simulink model "mbdo_full"  (Simulink 9.0)
settings: Solver=FixedStepDiscrete  StartTime=0  StopTime=simulationDuration  FixedStep=dt  MaxStep=0.001  RelTol=1e-3  EnableMultiTasking=on
InitFcn:
  | mbdoParams
StartFcn:
  | mbdoParams
values from neighbouring files (symbols this model uses):
  desBasePos = basePoseW    [mbdoParams.m]
undefined symbols (not defined in the file or in its folder): adjustEulerRates, computeFullDynamics, computeGrfs, computeVcross, DiscIntNeverNeededParam, Dj, dt, Gain, Ic, Kj, mapWrenchToTorques, q_des, simulinkAnim, updateStates
undefined symbols (not defined in the file): inputForce, Kdang, Kdlin, Kpang, Kplin
libraries: simulink x2
settings Model: SuppressorTable=22 serialization::archive 11 0 6 0 0 0 11 0  Creator=mfocchi  LastModifiedBy=nikhil
settings DataIOCC: LimitDataPoints=on
settings OptimizationCC: ExpressionDepthLimit=2147483647  InitFltsAndDblsToZero=on
settings DebuggingCC: SolverPrmCheckMsg=warning  FcnCallInpInsideContextMsg=warning  StateNameClashWarn=warning
settings GRTTargetCC: CombineOutputUpdateFcns=off  GRTInterface=on

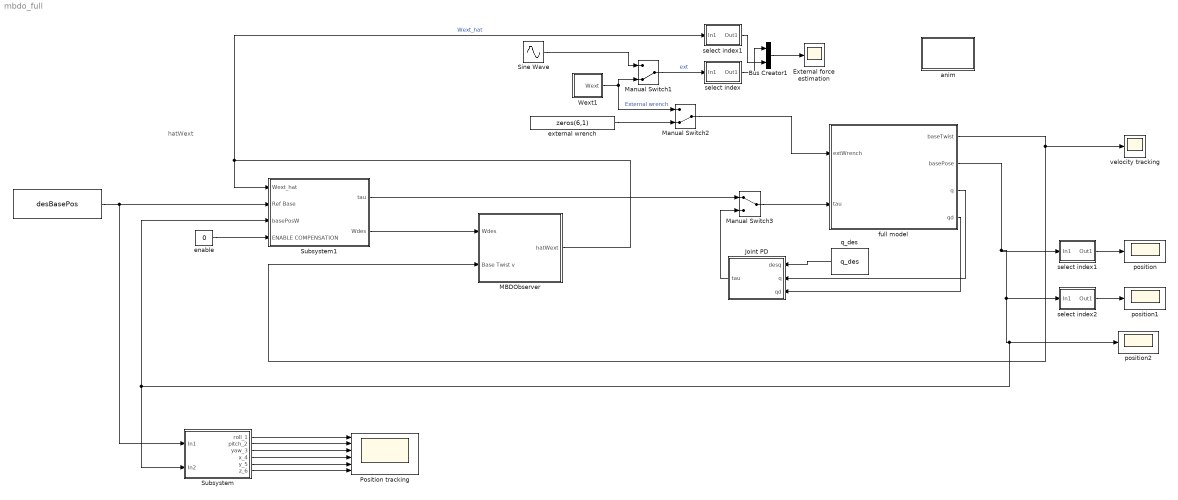
== system mbdo_full ==
  note: hatWext
  " " : Constant  Value=desBasePos
  Bus Creator1 : BusCreator  Inputs=2
  External force estimation : Scope
  Joint PD : Subsystem
  MBDObserver : Subsystem
  Manual Switch1 : ManualSwitch  CurrentSetting=0
  Manual Switch2 : ManualSwitch  CurrentSetting=0
  Manual Switch3 : ManualSwitch
  Position tracking : Scope  NumInputPorts=6
  Sine Wave : Sin  Amplitude=100  Frequency=2*pi*5  SampleTime=0
  Subsystem : Subsystem
  Subsystem1 : Subsystem
  Wext1 : Subsystem  mask{input=inputForce, fext=200, step_time=3}
  anim : Subsystem
  enable : Constant  Value=0
  external wrench : Constant  Value=zeros(6,1)
  full model : Subsystem
  position : Scope
  position1 : Scope
  position2 : Scope
  q_des : Constant  Value=q_des
  select index : Subsystem  mask{input=inputForce}
  select index1 : Subsystem  mask{input=6}
  "select index1 " : Subsystem  mask{input=inputForce}
  select index2 : Subsystem  mask{input=2}
  velocity tracking : Scope
  wires:
  " "/1 -> Subsystem/1(In1), Subsystem1/2(Ref Base)
  Bus Creator1/1 -> External force estimation/1
  select index/1(Out1) -> Bus Creator1/1
  "select index1 "/1(Out1) -> Bus Creator1/2
  Manual Switch1/1 -> select index/1(In1)  "ext"
  Wext1/1(Wext) -> Manual Switch1/2, Manual Switch2/1  "External wrench"
  Sine Wave/1 -> Manual Switch1/1
  full model/2(basePose) -> Subsystem1/3(basePosW), Subsystem/2(In2), position2/1, select index2/1(In1), select index1/1(In1)
  Subsystem/1(roll_1) -> Position tracking/1
  Subsystem/2(pitch_2) -> Position tracking/2
  Subsystem/3(yaw_3) -> Position tracking/3
  Subsystem/4(x_4) -> Position tracking/4
  Subsystem/5(y_5) -> Position tracking/5
  Subsystem/6(z_6) -> Position tracking/6
  MBDObserver/1("hatWext ") -> "select index1 "/1(In1), Subsystem1/1(Wext_hat)  "Wext_hat"
  full model/1(baseTwist) -> MBDObserver/2(Base Twist v), velocity tracking/1
  select index1/1(Out1) -> position/1
  external wrench/1 -> Manual Switch2/2
  Manual Switch2/1 -> full model/1(extWrench)
  Manual Switch3/1 -> full model/2(tau)
  q_des/1 -> Joint PD/1(desq)
  full model/3(q) -> Joint PD/2(q)
  Joint PD/1(tau) -> Manual Switch3/2
  select index2/1(Out1) -> position1/1
  full model/4(qd) -> Joint PD/3(qd)
  Subsystem1/2(Wdes) -> MBDObserver/1(Wdes)
  Subsystem1/1(tau) -> Manual Switch3/1
  enable/1 -> Subsystem1/4(ENABLE COMPENSATION)

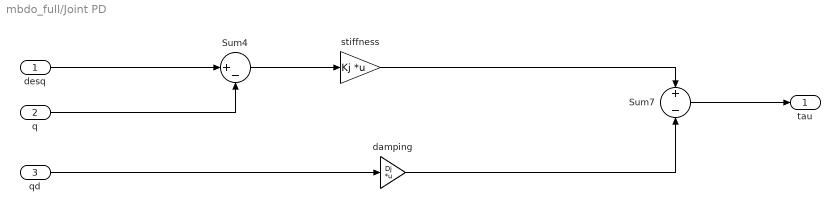
== system mbdo_full/Joint PD ==
  desq : Inport
  q : Inport  Port=2
  qd : Inport  Port=3
  Sum4 : Sum  Inputs=|+-
  Sum7 : Sum  Inputs=+|-
  damping : Gain  Gain=Dj  Multiplication=Matrix(K*u)
  stiffness : Gain  Gain=Kj  Multiplication=Matrix(K*u)
  tau : Outport
  wires:
  q/1 -> Sum4/2
  desq/1 -> Sum4/1
  Sum7/1 -> tau/1
  damping/1 -> Sum7/2
  stiffness/1 -> Sum7/1
  Sum4/1 -> stiffness/1
  qd/1 -> damping/1

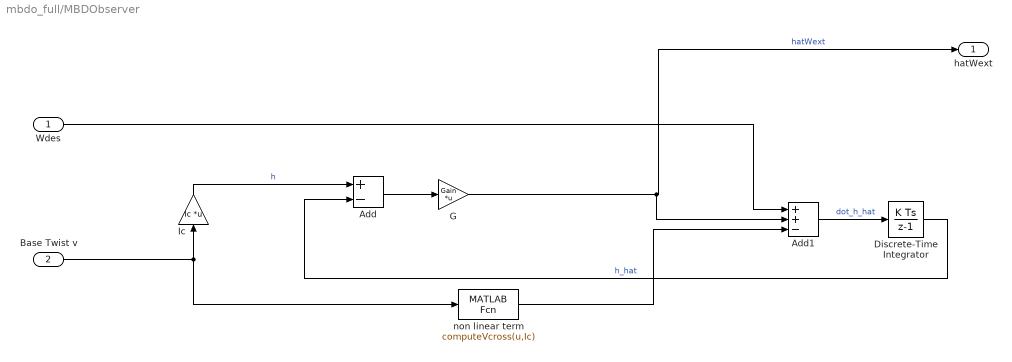
== system mbdo_full/MBDObserver ==
  Wdes : Inport
  Base Twist v : Inport  Port=2
  Add : Sum  Inputs=+-
  Add1 : Sum  Inputs=++-
  Discrete-Time Integrator : DiscreteIntegrator  InitialCondition=zeros(6,1)  InitialConditionSetting=State (most efficient)  SampleTime=dt  ICPrevOutput=DiscIntNeverNeededParam  ICPrevScaledInput=DiscIntNeverNeededParam
  G : Gain  Gain=Gain  Multiplication=Matrix(K*u)
  Ic : Gain  Gain=Ic  Multiplication=Matrix(K*u)
  non linear term : MATLABFcn  MATLABFcn=computeVcross(u,Ic)
  "hatWext " : Outport
  wires:
  G/1 -> Add1/2, "hatWext "/1  "hatWext"
  Wdes/1 -> Add1/1
  Base Twist v/1 -> non linear term/1, Ic/1
  Add/1 -> G/1
  Add1/1 -> Discrete-Time Integrator/1  "dot_h_hat"
  Ic/1 -> Add/1  "h"
  Discrete-Time Integrator/1 -> Add/2  "h_hat"
  non linear term/1 -> Add1/3

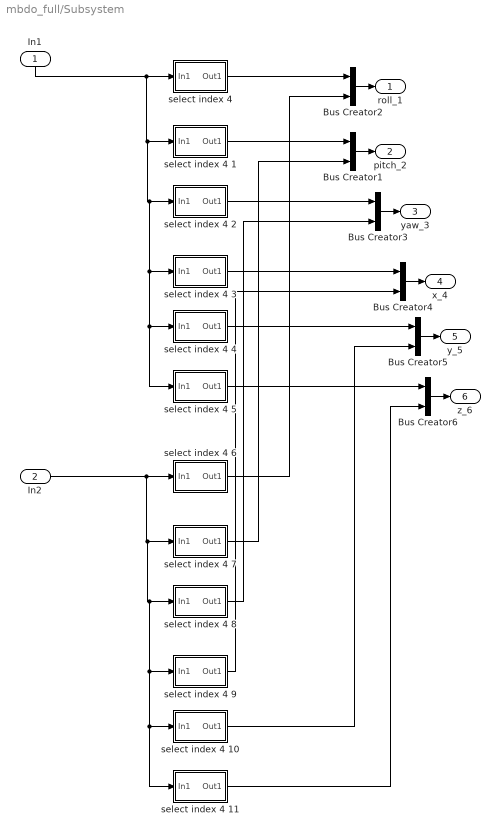
== system mbdo_full/Subsystem ==
  In1 : Inport
  In2 : Inport  Port=2
  Bus Creator{1..6} (6 alike) : BusCreator  Inputs=2
  "select index 4 " : Subsystem  mask{input=1}
  select index 4 1 : Subsystem  mask{input=2}
  select index 4 10 : Subsystem  mask{input=5}
  select index 4 11 : Subsystem  mask{input=6}
  select index 4 2 : Subsystem  mask{input=3}
  select index 4 3 : Subsystem  mask{input=4}
  select index 4 4 : Subsystem  mask{input=5}
  select index 4 5 : Subsystem  mask{input=6}
  select index 4 6 : Subsystem  mask{input=1}
  select index 4 7 : Subsystem  mask{input=2}
  select index 4 8 : Subsystem  mask{input=3}
  select index 4 9 : Subsystem  mask{input=4}
  roll_1 : Outport
  pitch_2 : Outport  Port=2
  yaw_3 : Outport  Port=3
  x_4 : Outport  Port=4
  y_5 : Outport  Port=5
  z_6 : Outport  Port=6
  wires:
  Bus Creator2/1 -> roll_1/1
  "select index 4 "/1(Out1) -> Bus Creator2/1
  In1/1 -> select index 4 5/1(In1), select index 4 4/1(In1), select index 4 3/1(In1), select index 4 2/1(In1), select index 4 1/1(In1), "select index 4 "/1(In1)
  In2/1 -> select index 4 11/1(In1), select index 4 10/1(In1), select index 4 9/1(In1), select index 4 8/1(In1), select index 4 7/1(In1), select index 4 6/1(In1)
  select index 4 6/1(Out1) -> Bus Creator2/2
  select index 4 7/1(Out1) -> Bus Creator1/2
  select index 4 1/1(Out1) -> Bus Creator1/1
  Bus Creator1/1 -> pitch_2/1
  Bus Creator3/1 -> yaw_3/1
  select index 4 8/1(Out1) -> Bus Creator3/2
  select index 4 9/1(Out1) -> Bus Creator4/2
  Bus Creator4/1 -> x_4/1
  Bus Creator5/1 -> y_5/1
  select index 4 10/1(Out1) -> Bus Creator5/2
  select index 4 11/1(Out1) -> Bus Creator6/2
  Bus Creator6/1 -> z_6/1
  select index 4 2/1(Out1) -> Bus Creator3/1
  select index 4 3/1(Out1) -> Bus Creator4/1
  select index 4 4/1(Out1) -> Bus Creator5/1
  select index 4 5/1(Out1) -> Bus Creator6/1

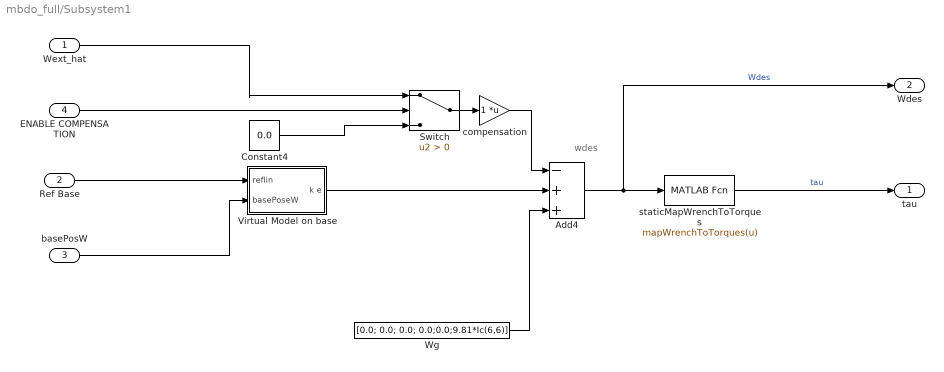
== system mbdo_full/Subsystem1 ==
  note: wdes
  Wext_hat : Inport
  Ref Base : Inport  Port=2
  basePosW : Inport  Port=3
  ENABLE COMPENSATION : Inport  Port=4
  Add4 : Sum  Inputs=-++
  Constant4 : Constant  Value=0.0
  Switch : Switch  Criteria=u2 > Threshold
  Virtual Model on base : Subsystem
  Wg : Constant  Value=[0.0; 0.0; 0.0; 0.0;0.0;9.81*Ic(6,6)]
  compensation : Gain  Multiplication=Matrix(K*u)
  staticMapWrenchToTorques : MATLABFcn  MATLABFcn=mapWrenchToTorques(u)
  tau : Outport
  Wdes : Outport  Port=2
  wires:
  basePosW/1 -> Virtual Model on base/2(basePoseW)
  Add4/1 -> Wdes/1, staticMapWrenchToTorques/1  "Wdes"
  Ref Base/1 -> Virtual Model on base/1(reflin)
  Constant4/1 -> Switch/3
  Switch/1 -> compensation/1
  Virtual Model on base/1(k e) -> Add4/2
  compensation/1 -> Add4/1
  Wg/1 -> Add4/3
  staticMapWrenchToTorques/1 -> tau/1  "tau"
  Wext_hat/1 -> Switch/1
  ENABLE COMPENSATION/1 -> Switch/2

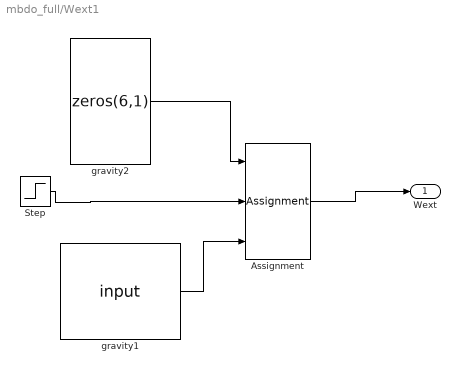
== system mbdo_full/Wext1 ==
  Assignment : Assignment  IndexOptions=Index vector (port)  Indices=1  OutputSizes=1
  Step : Step  Time=step_time  After=fext  SampleTime=0
  gravity1 : Constant  Value=input
  gravity2 : Constant  Value=zeros(6,1)
  Wext : Outport
  wires:
  Step/1 -> Assignment/2
  gravity2/1 -> Assignment/1
  gravity1/1 -> Assignment/3
  Assignment/1 -> Wext/1

== system mbdo_full/anim ==
  Constant1 : Constant  Value=0.0
  Terminator : Terminator
  anim : MATLABFcn  MATLABFcn=simulinkAnim()
  wires:
  anim/1 -> Terminator/1
  Constant1/1 -> anim/1

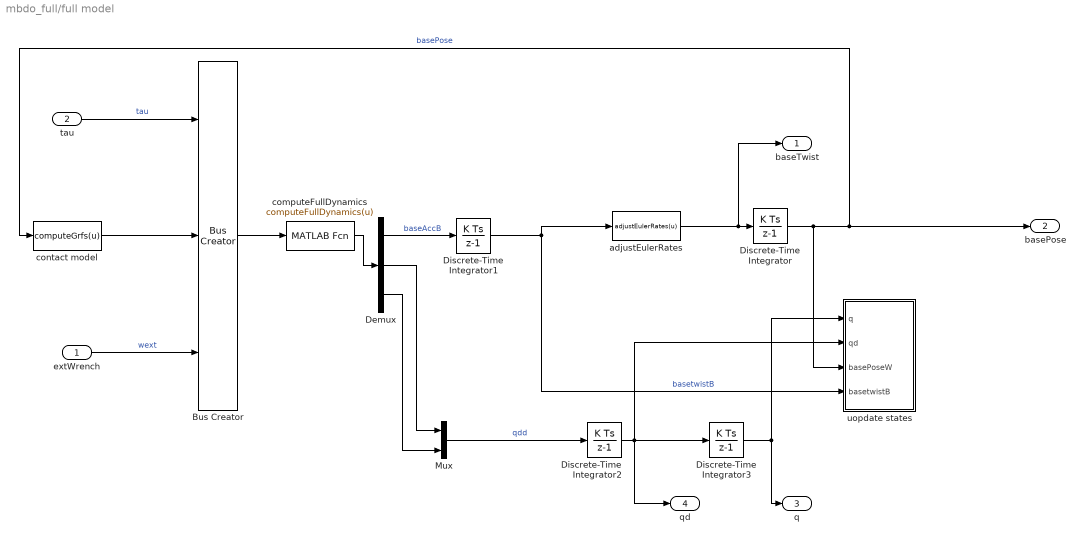
== system mbdo_full/full model ==
  extWrench : Inport
  tau : Inport  Port=2
  Bus Creator : BusCreator  Inputs=3
  Demux : Demux  Outputs=3
  Discrete-Time Integrator : DiscreteIntegrator  InitialCondition=desBasePos  InitialConditionSetting=State (most efficient)  SampleTime=dt  ICPrevOutput=DiscIntNeverNeededParam  ICPrevScaledInput=DiscIntNeverNeededParam
  Discrete-Time Integrator1 : DiscreteIntegrator  InitialCondition=zeros(6,1)  InitialConditionSetting=State (most efficient)  SampleTime=dt  ICPrevOutput=DiscIntNeverNeededParam  ICPrevScaledInput=DiscIntNeverNeededParam
  Discrete-Time Integrator2 : DiscreteIntegrator  InitialCondition=zeros(12,1)  InitialConditionSetting=State (most efficient)  SampleTime=dt  ICPrevOutput=DiscIntNeverNeededParam  ICPrevScaledInput=DiscIntNeverNeededParam
  Discrete-Time Integrator3 : DiscreteIntegrator  InitialCondition=q_des  InitialConditionSetting=State (most efficient)  SampleTime=dt  ICPrevOutput=DiscIntNeverNeededParam  ICPrevScaledInput=DiscIntNeverNeededParam
  Mux : Mux  Inputs=2
  adjustEulerRates : MATLABFcn  MATLABFcn=adjustEulerRates(u)  OutputDimensions=6
  computeFullDynamics : MATLABFcn  MATLABFcn=computeFullDynamics(u)  OutputDimensions=18
  contact model : MATLABFcn  MATLABFcn=computeGrfs(u)  OutputDimensions=12
  uopdate states : Subsystem
  baseTwist : Outport
  basePose : Outport  Port=2
  q : Outport  Port=3
  qd : Outport  Port=4
  wires:
  Bus Creator/1 -> computeFullDynamics/1
  Discrete-Time Integrator1/1 -> adjustEulerRates/1, uopdate states/4(basetwistB)  "basetwistB"
  tau/1 -> Bus Creator/1  "tau"
  extWrench/1 -> Bus Creator/3  "wext"
  computeFullDynamics/1 -> Demux/1
  Demux/1 -> Discrete-Time Integrator1/1  "baseAccB"
  Discrete-Time Integrator/1 -> uopdate states/3(basePoseW), contact model/1, basePose/1  "basePose"
  Demux/2 -> Mux/1
  Demux/3 -> Mux/2
  Discrete-Time Integrator2/1 -> qd/1, uopdate states/2(qd), Discrete-Time Integrator3/1
  Mux/1 -> Discrete-Time Integrator2/1  "qdd"
  Discrete-Time Integrator3/1 -> uopdate states/1(q), q/1
  adjustEulerRates/1 -> baseTwist/1, Discrete-Time Integrator/1
  contact model/1 -> Bus Creator/2

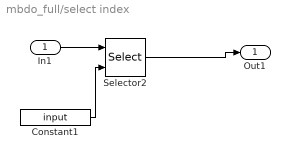
== system mbdo_full/select index ==
  In1 : Inport
  Constant1 : Constant  Value=input
  Selector2 : Selector  InputPortWidth=6  IndexOptions=Index vector (port)  Indices=[1 ]  OutputSizes=1
  Out1 : Outport
  wires:
  Constant1/1 -> Selector2/2
  In1/1 -> Selector2/1
  Selector2/1 -> Out1/1

== system mbdo_full/select index1 ==
  In1 : Inport
  Constant1 : Constant  Value=input
  Selector2 : Selector  InputPortWidth=6  IndexOptions=Index vector (port)  Indices=[1 ]  OutputSizes=1
  Out1 : Outport
  wires:
  Selector2/1 -> Out1/1
  In1/1 -> Selector2/1
  Constant1/1 -> Selector2/2

== system mbdo_full/select index1  ==
  In1 : Inport
  Constant1 : Constant  Value=input
  Selector2 : Selector  InputPortWidth=6  IndexOptions=Index vector (port)  Indices=[1 ]  OutputSizes=1
  Out1 : Outport
  wires:
  Selector2/1 -> Out1/1
  In1/1 -> Selector2/1
  Constant1/1 -> Selector2/2

== system mbdo_full/select index2 ==
  In1 : Inport
  Constant1 : Constant  Value=input
  Selector2 : Selector  InputPortWidth=6  IndexOptions=Index vector (port)  Indices=[1 ]  OutputSizes=1
  Out1 : Outport
  wires:
  Constant1/1 -> Selector2/2
  In1/1 -> Selector2/1
  Selector2/1 -> Out1/1

== system mbdo_full/Subsystem/select index 4  ==
  In1 : Inport
  Constant1 : Constant  Value=input
  Selector2 : Selector  InputPortWidth=6  IndexOptions=Index vector (port)  Indices=[1 ]  OutputSizes=1
  Out1 : Outport
  wires:
  Selector2/1 -> Out1/1
  In1/1 -> Selector2/1
  Constant1/1 -> Selector2/2

== system mbdo_full/Subsystem/select index 4 1 ==
  In1 : Inport
  Constant1 : Constant  Value=input
  Selector2 : Selector  InputPortWidth=6  IndexOptions=Index vector (port)  Indices=[1 ]  OutputSizes=1
  Out1 : Outport
  wires:
  Constant1/1 -> Selector2/2
  In1/1 -> Selector2/1
  Selector2/1 -> Out1/1

== system mbdo_full/Subsystem/select index 4 10 ==
  In1 : Inport
  Constant1 : Constant  Value=input
  Selector2 : Selector  InputPortWidth=6  IndexOptions=Index vector (port)  Indices=[1 ]  OutputSizes=1
  Out1 : Outport
  wires:
  Selector2/1 -> Out1/1
  In1/1 -> Selector2/1
  Constant1/1 -> Selector2/2

== system mbdo_full/Subsystem/select index 4 11 ==
  In1 : Inport
  Constant1 : Constant  Value=input
  Selector2 : Selector  InputPortWidth=6  IndexOptions=Index vector (port)  Indices=[1 ]  OutputSizes=1
  Out1 : Outport
  wires:
  Constant1/1 -> Selector2/2
  In1/1 -> Selector2/1
  Selector2/1 -> Out1/1

== system mbdo_full/Subsystem/select index 4 2 ==
  In1 : Inport
  Constant1 : Constant  Value=input
  Selector2 : Selector  InputPortWidth=6  IndexOptions=Index vector (port)  Indices=[1 ]  OutputSizes=1
  Out1 : Outport
  wires:
  Selector2/1 -> Out1/1
  In1/1 -> Selector2/1
  Constant1/1 -> Selector2/2

== system mbdo_full/Subsystem/select index 4 3 ==
  In1 : Inport
  Constant1 : Constant  Value=input
  Selector2 : Selector  InputPortWidth=6  IndexOptions=Index vector (port)  Indices=[1 ]  OutputSizes=1
  Out1 : Outport
  wires:
  Constant1/1 -> Selector2/2
  In1/1 -> Selector2/1
  Selector2/1 -> Out1/1

== system mbdo_full/Subsystem/select index 4 4 ==
  In1 : Inport
  Constant1 : Constant  Value=input
  Selector2 : Selector  InputPortWidth=6  IndexOptions=Index vector (port)  Indices=[1 ]  OutputSizes=1
  Out1 : Outport
  wires:
  Selector2/1 -> Out1/1
  In1/1 -> Selector2/1
  Constant1/1 -> Selector2/2

== system mbdo_full/Subsystem/select index 4 5 ==
  In1 : Inport
  Constant1 : Constant  Value=input
  Selector2 : Selector  InputPortWidth=6  IndexOptions=Index vector (port)  Indices=[1 ]  OutputSizes=1
  Out1 : Outport
  wires:
  Constant1/1 -> Selector2/2
  In1/1 -> Selector2/1
  Selector2/1 -> Out1/1

== system mbdo_full/Subsystem/select index 4 6 ==
  In1 : Inport
  Constant1 : Constant  Value=input
  Selector2 : Selector  InputPortWidth=6  IndexOptions=Index vector (port)  Indices=[1 ]  OutputSizes=1
  Out1 : Outport
  wires:
  Selector2/1 -> Out1/1
  In1/1 -> Selector2/1
  Constant1/1 -> Selector2/2

== system mbdo_full/Subsystem/select index 4 7 ==
  In1 : Inport
  Constant1 : Constant  Value=input
  Selector2 : Selector  InputPortWidth=6  IndexOptions=Index vector (port)  Indices=[1 ]  OutputSizes=1
  Out1 : Outport
  wires:
  Constant1/1 -> Selector2/2
  In1/1 -> Selector2/1
  Selector2/1 -> Out1/1

== system mbdo_full/Subsystem/select index 4 8 ==
  In1 : Inport
  Constant1 : Constant  Value=input
  Selector2 : Selector  InputPortWidth=6  IndexOptions=Index vector (port)  Indices=[1 ]  OutputSizes=1
  Out1 : Outport
  wires:
  Selector2/1 -> Out1/1
  In1/1 -> Selector2/1
  Constant1/1 -> Selector2/2

== system mbdo_full/Subsystem/select index 4 9 ==
  In1 : Inport
  Constant1 : Constant  Value=input
  Selector2 : Selector  InputPortWidth=6  IndexOptions=Index vector (port)  Indices=[1 ]  OutputSizes=1
  Out1 : Outport
  wires:
  Constant1/1 -> Selector2/2
  In1/1 -> Selector2/1
  Selector2/1 -> Out1/1

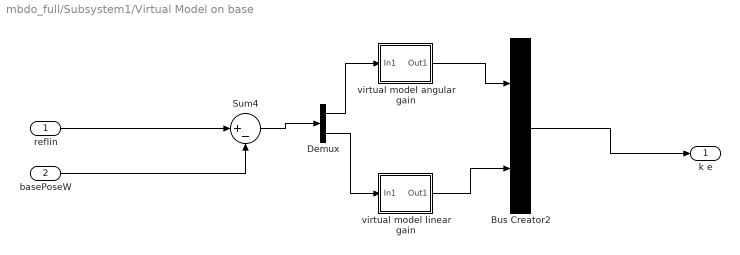
== system mbdo_full/Subsystem1/Virtual Model on base ==
  reflin : Inport
  basePoseW : Inport  Port=2
  Bus Creator2 : BusCreator  Inputs=2
  Demux : Demux  Outputs=2
  Sum4 : Sum  Inputs=|+-
  virtual model angular gain : Subsystem  mask{stiffness=Kpang, damping=Kdang}
  virtual model linear gain : Subsystem  mask{stiffness=Kplin, damping=Kdlin}
  k e : Outport
  wires:
  Demux/2 -> virtual model linear gain/1(In1)
  Sum4/1 -> Demux/1
  Demux/1 -> virtual model angular gain/1(In1)
  virtual model linear gain/1(Out1) -> Bus Creator2/2
  virtual model angular gain/1(Out1) -> Bus Creator2/1
  basePoseW/1 -> Sum4/2
  Bus Creator2/1 -> k e/1
  reflin/1 -> Sum4/1

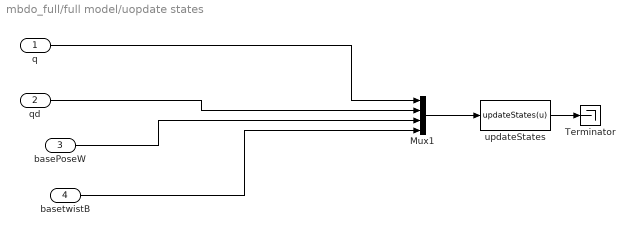
== system mbdo_full/full model/uopdate states ==
  q : Inport
  qd : Inport  Port=2
  basePoseW : Inport  Port=3
  basetwistB : Inport  Port=4
  Mux1 : Mux
  Terminator : Terminator
  updateStates : MATLABFcn  MATLABFcn=updateStates(u)
  wires:
  basePoseW/1 -> Mux1/3
  basetwistB/1 -> Mux1/4
  qd/1 -> Mux1/2
  Mux1/1 -> updateStates/1
  updateStates/1 -> Terminator/1
  q/1 -> Mux1/1

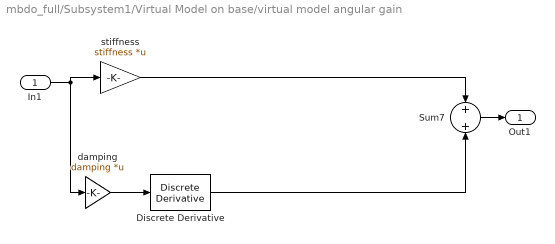
== system mbdo_full/Subsystem1/Virtual Model on base/virtual model angular gain ==
  In1 : Inport
  Discrete Derivative : simulink/Discrete/Discrete Derivative  gainval=1.0  ICPrevScaledInput=0.0  OutMin=[]  OutMax=[]  OutDataType=fixdt(1, 16)  OutScaling=2^-10  DoSatur=off
  Sum7 : Sum  Inputs=+|+
  damping : Gain  Gain=damping  Multiplication=Matrix(K*u)
  stiffness : Gain  Gain=stiffness  Multiplication=Matrix(K*u)
  Out1 : Outport
  wires:
  Sum7/1 -> Out1/1
  In1/1 -> stiffness/1, damping/1
  stiffness/1 -> Sum7/1
  damping/1 -> Discrete Derivative/1
  Discrete Derivative/1 -> Sum7/2

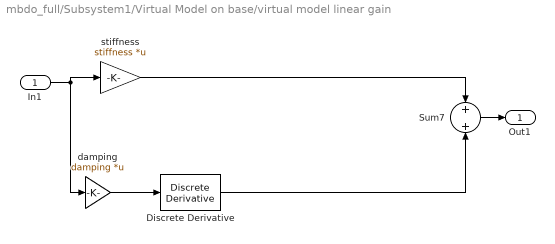
== system mbdo_full/Subsystem1/Virtual Model on base/virtual model linear gain ==
  In1 : Inport
  Discrete Derivative : simulink/Discrete/Discrete Derivative  gainval=1.0  ICPrevScaledInput=0.0  OutMin=[]  OutMax=[]  OutDataType=fixdt(1, 16)  OutScaling=2^-10  DoSatur=off
  Sum7 : Sum  Inputs=+|+
  damping : Gain  Gain=damping  Multiplication=Matrix(K*u)
  stiffness : Gain  Gain=stiffness  Multiplication=Matrix(K*u)
  Out1 : Outport
  wires:
  stiffness/1 -> Sum7/1
  In1/1 -> damping/1, stiffness/1
  Sum7/1 -> Out1/1
  damping/1 -> Discrete Derivative/1
  Discrete Derivative/1 -> Sum7/2
